simulink model "TestCHBModule"  (R2025b)
settings: Solver=ode23t  StartTime=0.0  StopTime=5  FixedStep=50e-6  RelTol=1e-3
libraries: fl_lib x8, nesl_utility x5, datacenter_lib x1, slpidlib x1
settings Model: Creator=saprasad  LastModifiedBy=saprasad
settings SimscapeCC: ExplicitSolverDiagnosticOptions=none  SimscapeLogType=all

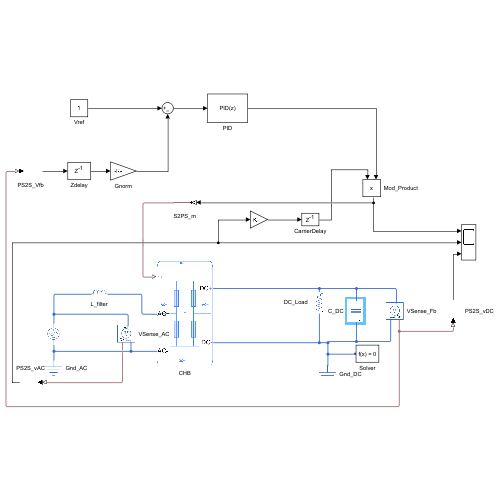
[thumbnail: Simulink's stored preview of the top-level diagram]
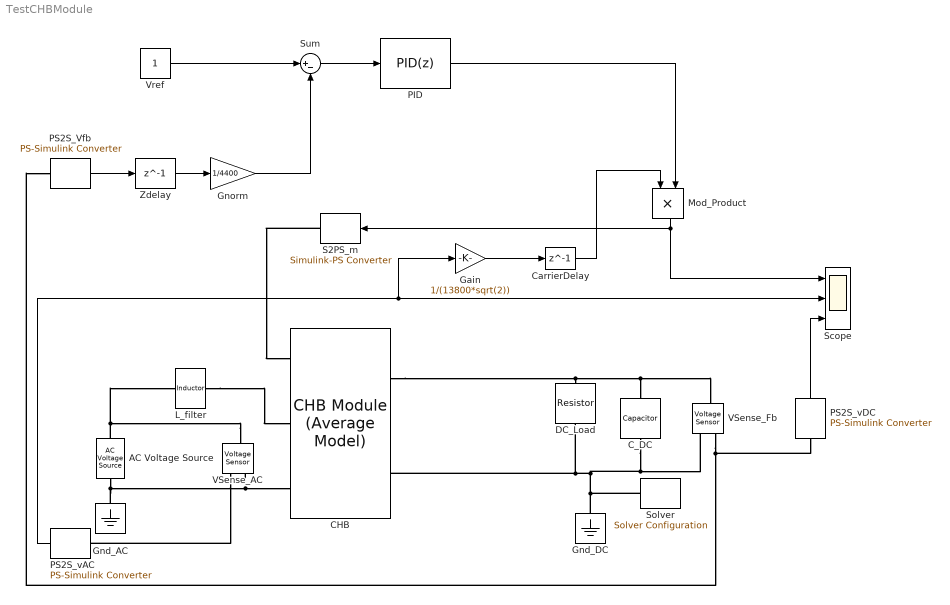
== system TestCHBModule ==
  AC Voltage Source : fl_lib/Electrical/Electrical Sources/AC Voltage Source  amp=13800 V  shift=0 deg  frequency=60 Hz
  CHB : datacenter_lib/CHB Module (Average Model)  OnResistance=1e-6 Ohm  GridVoltage=13800 V  TotalDCVoltage=13200 V  iAC_specify=off  iAC_priority=None  iAC=0 A  iAC_nominal_specify=off  iAC_nominal_value=1  iAC_nominal_unit=A  vAC_specify=off  vAC_priority=None  vAC=0 V  vAC_nominal_specify=off  vAC_nominal_value=1  vAC_nominal_unit=V  iDC_specify=off  iDC_priority=None  iDC=0 A  iDC_nominal_specify=off  iDC_nominal_value=1  iDC_nominal_unit=A  vDC_specify=off  vDC_priority=None  vDC=0 V  vDC_nominal_specify=off  vDC_nominal_value=1  vDC_nominal_unit=V  vOn_specify=off  vOn_priority=None  vOn=0 V  vOn_nominal_specify=off  vOn_nominal_value=1  vOn_nominal_unit=V
      settings: InternalSimscapePortConfiguration="{\"Bottom\":[],\"Left\":[{\"id\":\"m\",\"label\":\"m\",\"type\":\"input\"},{\"id\":\"ACPositive\",\"label\":\"AC+\",\"type\":\"foundation.electrical.electrical\"},{\"id\":\"ACNegative\",\"label\":\"AC-\",\"type\":\"foundation.electrical.electrical\"}],\"Right\":[{\"id\":\"DCPositive\",\"label\":\"DC+\",\"type\":\"foundation.electrical.electrical\"},{\"id\":\"DCNegative\",\"label\":\"DC-\",\"type\":\"foundation.electrical.electrical\"}],\"Top\":[]}"
  C_DC : fl_lib/Electrical/Electrical Elements/Capacitor  c=1 F  r=1e-6 Ohm  g=0 1/Ohm  i_specify=off  i_priority=None  i=0 A  i_nominal_specify=off  i_nominal_value=1  i_nominal_unit=A  v_specify=off  v_priority=None  v=0 V  v_nominal_specify=off  v_nominal_value=1  v_nominal_unit=V  vc_specify=on  vc_priority=High  vc=4400 V  vc_nominal_specify=off  vc_nominal_value=1  vc_nominal_unit=V
  CarrierDelay : Delay  DelayLength=1  SampleTime=50e-6
  DC_Load : fl_lib/Electrical/Electrical Elements/Resistor  R=100 Ohm  i_specify=off  i_priority=None  i=0 A  i_nominal_specify=off  i_nominal_value=1  i_nominal_unit=A  v_specify=off  v_priority=None  v=0 V  v_nominal_specify=off  v_nominal_value=1  v_nominal_unit=V
  Gain : Gain  Gain=1/(13800*sqrt(2))
  Gnd_AC : fl_lib/Electrical/Electrical Elements/Electrical Reference
  Gnd_DC : fl_lib/Electrical/Electrical Elements/Electrical Reference
  Gnorm : Gain  Gain=1/4400
  L_filter : fl_lib/Electrical/Electrical Elements/Inductor  l=5e-3 H  r=0.1 Ohm  g=1e-9 1/Ohm  i_specify=off  i_priority=None  i=0 A  i_nominal_specify=off  i_nominal_value=1  i_nominal_unit=A  v_specify=off  v_priority=None  v=0 V  v_nominal_specify=off  v_nominal_value=1  v_nominal_unit=V  i_L_specify=off  i_L_priority=High  i_L=0 A  i_L_nominal_specify=off  i_L_nominal_value=1  i_L_nominal_unit=A
  Mod_Product : Product
  PID : slpidlib/PID Controller  Controller=PID  Form=Parallel  TimeDomain=Discrete-time  UseExternalTs=off  SampleTime=50e-6  IntegratorMethod=Forward Euler  FilterMethod=Forward Euler  ControllerParametersSource=internal  P=100  I=800  UseKiTs=off  D=0  UseExternalDerivativeSource=off  N=100  UseFilter=on  TunerSelectOption=Transfer Function Based (PID Tuner App)  InitialConditionSource=internal  InitialConditionForIntegrator=0  InitialConditionForFilter=0  DifferentiatorICPrevScaledInput=0  ExternalReset=none  TrackingMode=off  Kt=1  LimitOutput=off  SatLimitsSource=internal  UpperSaturationLimit=inf  LowerSaturationLimit=-inf  LinearizeAsGain=off  AntiWindupMode=none  Kb=1  LimitIntegrator=off  UpperIntegratorSaturationLimit=inf  LowerIntegratorSaturationLimit=-inf  POutMin=[]  POutMax=[]  IOutMin=[]  IOutMax=[]  DOutMin=[]  DOutMax=[]  NOutMin=[]  NOutMax=[]  SumOutMin=[]  SumOutMax=[]  SaturationOutMin=[]  SaturationOutMax=[]  PParamMin=[]  PParamMax=[]  IParamMin=[]  IParamMax=[]  DParamMin=[]  DParamMax=[]  NParamMin=[]  NParamMax=[]  KbParamMin=[]  KbParamMax=[]  KtParamMin=[]  KtParamMax=[]  KbOutMin=[]  KbOutMax=[]  KtOutMin=[]  KtOutMax=[]  IntegratorOutMin=[]  IntegratorOutMax=[]  FilterOutMin=[]  FilterOutMax=[]  SumI1OutMin=[]  SumI1OutMax=[]  SumI2OutMin=[]  SumI2OutMax=[]  SumI3OutMin=[]  SumI3OutMax=[]  SumI4OutMin=[]  SumI4OutMax=[]  SumDOutMin=[]  SumDOutMax=[]  DifferentiatorOutMin=[]  DifferentiatorOutMax=[]  FilterDiffOutCoefMin=[]  FilterDiffOutCoefMax=[]  ReciprocalOutMin=[]  ReciprocalOutMax=[]  SumDenOutMin=[]  SumDenOutMax=[]  SumNumOutMin=[]  SumNumOutMax=[]  DivideOutMin=[]  DivideOutMax=[]  UdiffTsProdOutMin=[]  UdiffTsProdOutMax=[]  NTsProdOutMin=[]  NTsProdOutMax=[]  UintegralTsProdOutMin=[]  UintegralTsProdOutMax=[]  UngainTsProdOutMin=[]  UngainTsProdOutMax=[]  ClampingZeroOutDataTypeStr=Inherit: Inherit via back propagation  ClampingZeroOutMin=[]  ClampingZeroOutMax=[]  FilterDenConstantOutDataTypeStr=Inherit: Inherit via back propagation  FilterDenConstantOutMin=[]  FilterDenConstantOutMax=[]  PCopyOutDataTypeStr=Inherit: Inherit via back propagation  PCopyOutMin=[]  PCopyOutMax=[]  NCopyOutDataTypeStr=Inherit: Inherit via back propagation  NCopyOutMin=[]  NCopyOutMax=[]  IntegratorContinuousStateAttributes=''  IntegratorStateMustResolveToSignalObject=off  IntegratorRTWStateStorageClass=Auto  FilterContinuousStateAttributes=''  FilterStateMustResolveToSignalObject=off  FilterRTWStateStorageClass=Auto  ParallelPVariant=InternalParameters  IdealPVariant=Disabled  IVariant=InternalParameters  DVariant=InternalParameters  IntegratorVariant=Discrete  SatVariant=Disabled  AWVariant=Passthrough  PCopyVariant=Disabled  TRVariant=Disabled  FdbkBlocksVariant=Forward  IdealPFdbkVariant=Disabled  SatFdbkVariant=Disabled  DerivativeFilterVariant=ForwardEulerFilter  NVariant=InternalParameters  NCopyVariant=Disabled  FilterICVariant=InternalICsFilter  IntegratorICVariant=InternalICs  ExternalResetVariant=Disabled  TRSumVariant=Passthrough  SumFdbkVariant=Disabled  SumVariant=Sum_PID  TsampFilterVariant=InternalTs  TsampNgainVariant=Passthrough  TsampIntegralVariant=Disabled_SignalSpec  ExternalSaturationOutDataTypeStr=Inherit: Same as second input  DerivativeSourceVariant=ErrorSignal  PreIntVariant=InternalPreInt
      settings: LibrarySourceBlock=simulink/Discrete/Discrete PID Controller
  PS2S_Vfb : nesl_utility/PS-Simulink Converter  PhysicalDomain=network_engine_domain  SubClassName=ps_output  LeftPortType=input  RightPortType=output  PseudoPeriodic=off  Frequencies=[]  VectorFormat=inherit  Unit=inherit  AffineConversion=off
  PS2S_vAC : nesl_utility/PS-Simulink Converter  PhysicalDomain=network_engine_domain  SubClassName=ps_output  LeftPortType=input  RightPortType=output  PseudoPeriodic=off  Frequencies=[]  VectorFormat=inherit  Unit=inherit  AffineConversion=off
  PS2S_vDC : nesl_utility/PS-Simulink Converter  PhysicalDomain=network_engine_domain  SubClassName=ps_output  LeftPortType=input  RightPortType=output  PseudoPeriodic=off  Frequencies=[]  VectorFormat=inherit  Unit=inherit  AffineConversion=off
  S2PS_m : nesl_utility/Simulink-PS Converter  PhysicalDomain=network_engine_domain  SubClassName=ps_input  LeftPortType=input  RightPortType=output  PseudoPeriodic=off  Frequencies=[]  NoiseDistribution=none  NoiseParameters=[]  Unit=1  AffineConversion=off  FilteringAndDerivatives=filter  SimscapeFilterOrder=1  InputFilterTimeConstant=1e-3  UdotUserProvided=0
  Scope : Scope  NumInputPorts=3
      settings: ActiveDisplayYMinimum=-17215.961065388085  ActiveDisplayYMaximum=17215.961065388045
  Solver : nesl_utility/Solver Configuration  PhysicalDomain=network_engine_domain  SubClassName=solver  LeftPortType=input  RightPortType=generic  Tones=[]  Harmonics=[]  SimulateNoise=off  Profile=off  UseLocalSampling=off  EnableSwitchedLinearOptims=on  FrequencyDomain=off  UseCCode=off  RelTol=0.001  AbsTol=0.001  MinStep=1e-09  ToWorkspace=off  RevertToSquareIcSolve=off  NumHomotopyIterations=100  PhasorMode=off  PhasorModeNumHarmonics=1  ConsistencySolver=NEWTON_XTOL_AFTER_FTOL  IndexReductionMethod=DerivativeReplacement  DoDC=off  ResidualTolerance=1e-09  ConsistencyTolSource=GLOBAL  ConsistencyAbsTol=0.001  ConsistencyRelTol=0.001  ConsistencyTolFactor=0.001  UseLocalSolver=on  LocalSolverChoice=NE_BACKWARD_EULER_ADVANCER  ResolveIndetEquations=off  FunctionEvalNumThread=1  LocalSolverSampleTime=0.001  DoFixedCost=off  MaxNonlinIter=3  MaxModeIter=2  ComputeImpulses=off  ImpulseIterations=2  LinearAlgebra=auto  LinearAlgebraNumThread=0  EquationFormulation=NE_TIME_EF  DelaysMemoryBudget=1024  AutomaticFiltering=off  FilteringTimeConstant=0.001  PartitionStorageMethod=AS_NEEDED  PartitionMemoryBudget=1024  PartitionMethod=ROBUST  MultibodyUseLocalSolver=off  MultibodyLocalSolverChoice=ODE1  MultibodyLocalSolverSampleTime=0.001
  Sum : Sum  Inputs=|+-
  VSense_AC : fl_lib/Electrical/Electrical Sensors/Voltage Sensor
  VSense_Fb : fl_lib/Electrical/Electrical Sensors/Voltage Sensor
  Vref : Constant
  Zdelay : Delay  DelayLength=1  InitialCondition=0  SampleTime=50e-6
  wires:
  PS2S_vAC/1 -> Scope/2, Gain/1
  PS2S_vDC/1 -> Scope/3
  Vref/1 -> Sum/1
  Zdelay/1 -> Gnorm/1
  PS2S_Vfb/1 -> Zdelay/1
  Sum/1 -> PID/1
  Gnorm/1 -> Sum/2
  Mod_Product/1 -> Scope/1, S2PS_m/1
  Gain/1 -> CarrierDelay/1
  CarrierDelay/1 -> Mod_Product/1
  PID/1 -> Mod_Product/2
  connections:
  VSense_AC/RConn1 -- PS2S_vAC/LConn1
  S2PS_m/RConn1 -- CHB/LConn1
  VSense_Fb/RConn1 -- PS2S_Vfb/LConn1 -- PS2S_vDC/LConn1
  C_DC/RConn1 -- Solver/RConn1 -- Gnd_DC/LConn1 -- DC_Load/RConn1 -- CHB/RConn2 -- VSense_Fb/RConn2
  Gnd_AC/LConn1 -- AC Voltage Source/RConn1 -- VSense_AC/RConn2 -- CHB/LConn3
  CHB/RConn1 -- DC_Load/LConn1 -- VSense_Fb/LConn1 -- C_DC/LConn1
  VSense_AC/LConn1 -- AC Voltage Source/LConn1 -- L_filter/LConn1
  L_filter/RConn1 -- CHB/LConn2
